simulink model "shred_mem_test"  (R2022b)
settings: Solver=VariableStepAuto  StartTime=0.0  StopTime=inf  RelTol=1e-3
settings Model: Creator=emu  LastModifiedBy=emu

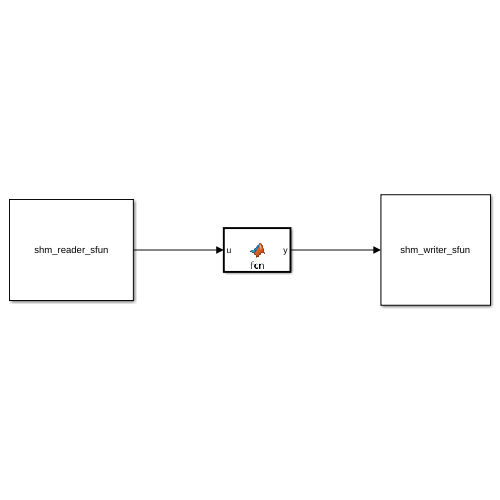
[thumbnail: Simulink's stored preview of the top-level diagram]
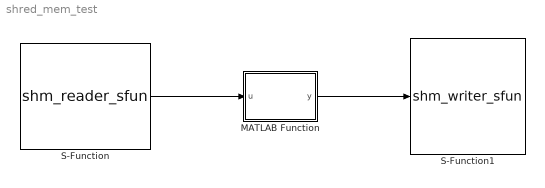
== system shred_mem_test ==
  MATLAB Function : MATLAB Function  TreatAsAtomicUnit=on
  S-Function : S-Function  FunctionName=shm_reader_sfun  Parameters='/my_custom_shm_read'  SFunctionDeploymentMode=off  EnableBusSupport=off
  S-Function1 : S-Function  FunctionName=shm_writer_sfun  Parameters='my_custom_shm_write'  SFunctionDeploymentMode=off  EnableBusSupport=off
  wires:
  S-Function/1 -> MATLAB Function/1(u)
  MATLAB Function/1(y) -> S-Function1/1

== matlab function shred_mem_test/MATLAB Function ==
  settings: updateMethod=DISCRETE  sampleTime=1e-3
  data: u input; y output
function y = fcn(u)

y = u(1:100);
